simulink model "stopien_swobody"  (R2024b)
settings: Solver=VariableStepAuto  StartTime=0.0  StopTime=10.0  RelTol=1e-3
undefined symbols (not defined in the file): Amp, c, f, k, m
settings Model: Creator=user  LastModifiedBy=jakub

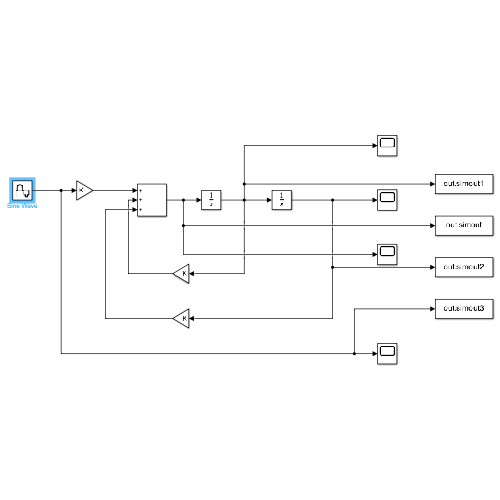
[thumbnail: Simulink's stored preview of the top-level diagram]
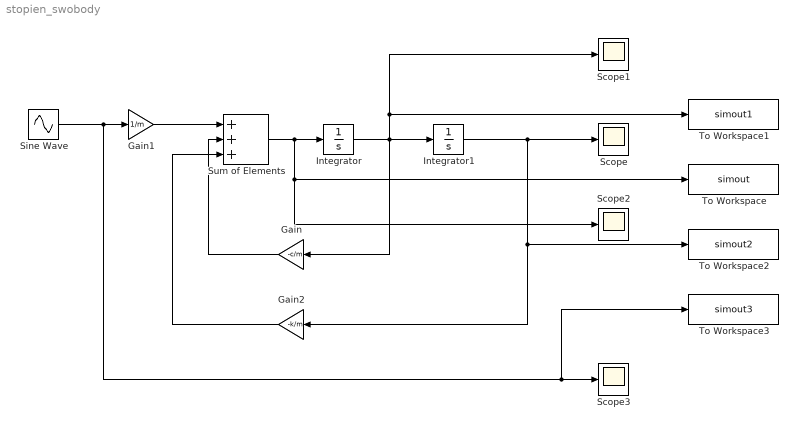
== system stopien_swobody ==
  Gain : Gain  Gain=-c/m
  Gain1 : Gain  Gain=1/m
  Gain2 : Gain  Gain=-k/m
  Integrator : Integrator
  Integrator1 : Integrator
  Scope{,1..3} (4 alike) : Scope
  Sine Wave : Sin  Amplitude=Amp  Frequency=2*pi*f  SampleTime=0.001
  Sum of Elements : Sum  Inputs=+++
  To Workspace : ToWorkspace  VariableName=simout  SaveFormat=Structure  SampleTime=-1
  To Workspace1 : ToWorkspace  VariableName=simout1  SaveFormat=Structure  SampleTime=-1
  To Workspace2 : ToWorkspace  VariableName=simout2  SaveFormat=Structure  SampleTime=-1
  To Workspace3 : ToWorkspace  VariableName=simout3  SaveFormat=Structure  SampleTime=-1
  wires:
  Sine Wave/1 -> To Workspace3/1, Scope3/1, Gain1/1
  Gain1/1 -> Sum of Elements/1
  Gain/1 -> Sum of Elements/2
  Gain2/1 -> Sum of Elements/3
  Sum of Elements/1 -> Scope2/1, To Workspace/1, Integrator/1
  Integrator/1 -> To Workspace1/1, Scope1/1, Gain/1, Integrator1/1
  Integrator1/1 -> To Workspace2/1, Gain2/1, Scope/1
